simulink library "sm_excv_scene_lib"  (R2023a)
settings: Solver=VariableStepAuto  StartTime=0.0  StopTime=10.0  RelTol=1e-3
undefined symbols (not defined in the file): B1, B2, B3, B4, B5, B6, B7, B8, Excv, L1, L2, L3, L4, L5, L6, L7, L8, L9, Road, S1, S2, Scene, Scene_Data, SceneData, X, Y, Z
libraries: sm_lib x65, sm_tracked_vehicle_lib x47, $bdroot x45, nesl_utility x10
(part 3 of 3)

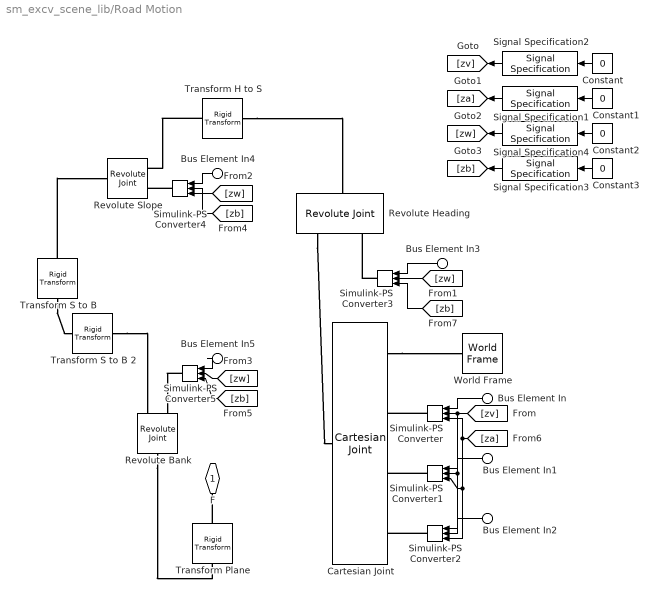
== system sm_excv_scene_lib/Road Motion ==
  Bus Element In : Inport  PortName=Road  Element=px
  Bus Element In1 : Inport  PortName=Road  Element=py
  Bus Element In2 : Inport  PortName=Road  Element=pz
  Bus Element In3 : Inport  PortName=Road  Element=qz
  Bus Element In4 : Inport  PortName=Road  Element=qy
  Bus Element In5 : Inport  PortName=Road  Element=qx
  Cartesian Joint : sm_lib/Joints/Cartesian Joint  JointMode=Normal  SenseConstraintForce=off  SenseConstraintForceX=off  SenseConstraintForceY=off  SenseConstraintForceZ=off  SenseConstraintTorque=off  SenseConstraintTorqueX=off  SenseConstraintTorqueY=off  SenseConstraintTorqueZ=off  SenseTotalForce=off  SenseTotalForceX=off  SenseTotalForceY=off  SenseTotalForceZ=off  SenseTotalTorque=off  SenseTotalTorqueX=off  SenseTotalTorqueY=off  SenseTotalTorqueZ=off  CompositeWrenchDir=FollowerOnBase  CompositeWrenchFrame=BaseFrame  PxEquilibriumPosition=0  PxEquilibriumPositionUnits=m  PxSpringStiffness=0  PxSpringStiffnessUnits=N/m  PxDampingCoefficient=0  PxDampingCoefficientUnits=N/(m/s)  PxTorqueActuationMode=ComputedTorque  PxMotionActuationMode=InputMotion  PxSensePosition=off  PxSenseVelocity=off  PxSenseAcceleration=off  PxSenseTorqueForce=off  PxSenseLowerLimitTorqueForce=off  PxSenseUpperLimitTorqueForce=off  PxLowerLimitSpecify=off  PxLowerLimitBound=-1  PxLowerLimitBoundUnits=m  PxLowerLimitStiffness=1e6  PxLowerLimitStiffnessUnits=N/m  PxLowerLimitDamping=1e3  PxLowerLimitDampingUnits=N/(m/s)  PxLowerLimitTransitionRegionWidth=1e-4  PxLowerLimitTransitionRegionWidthUnits=m  PxUpperLimitSpecify=off  PxUpperLimitBound=1  PxUpperLimitBoundUnits=m  PxUpperLimitStiffness=1e6  PxUpperLimitStiffnessUnits=N/m  PxUpperLimitDamping=1e3  PxUpperLimitDampingUnits=N/(m/s)  PxUpperLimitTransitionRegionWidth=1e-4  PxUpperLimitTransitionRegionWidthUnits=m  PxPositionTargetSpecify=off  PxPositionTargetPriority=High  PxPositionTargetValue=0  PxPositionTargetValueUnits=m  PxVelocityTargetSpecify=off  PxVelocityTargetPriority=High  PxVelocityTargetValue=0  PxVelocityTargetValueUnits=m/s  PyEquilibriumPosition=0  PyEquilibriumPositionUnits=m  PySpringStiffness=0  PySpringStiffnessUnits=N/m  PyDampingCoefficient=0  PyDampingCoefficientUnits=N/(m/s)  PyTorqueActuationMode=ComputedTorque  PyMotionActuationMode=InputMotion  PySensePosition=off  PySenseVelocity=off  PySenseAcceleration=off  PySenseTorqueForce=off  PySenseLowerLimitTorqueForce=off  PySenseUpperLimitTorqueForce=off  PyLowerLimitSpecify=off  PyLowerLimitBound=-1  PyLowerLimitBoundUnits=m  PyLowerLimitStiffness=1e6  PyLowerLimitStiffnessUnits=N/m  PyLowerLimitDamping=1e3  PyLowerLimitDampingUnits=N/(m/s)  PyLowerLimitTransitionRegionWidth=1e-4  PyLowerLimitTransitionRegionWidthUnits=m  PyUpperLimitSpecify=off  PyUpperLimitBound=1  PyUpperLimitBoundUnits=m  PyUpperLimitStiffness=1e6  PyUpperLimitStiffnessUnits=N/m  PyUpperLimitDamping=1e3  PyUpperLimitDampingUnits=N/(m/s)  PyUpperLimitTransitionRegionWidth=1e-4  PyUpperLimitTransitionRegionWidthUnits=m  PyPositionTargetSpecify=off  PyPositionTargetPriority=High  PyPositionTargetValue=0  PyPositionTargetValueUnits=m  PyVelocityTargetSpecify=off  PyVelocityTargetPriority=High  PyVelocityTargetValue=0  PyVelocityTargetValueUnits=m/s  PzEquilibriumPosition=0  PzEquilibriumPositionUnits=m  PzSpringStiffness=0  PzSpringStiffnessUnits=N/m  PzDampingCoefficient=0  PzDampingCoefficientUnits=N/(m/s)  PzTorqueActuationMode=ComputedTorque  PzMotionActuationMode=InputMotion  PzSensePosition=off  PzSenseVelocity=off  PzSenseAcceleration=off  PzSenseTorqueForce=off  PzSenseLowerLimitTorqueForce=off  PzSenseUpperLimitTorqueForce=off  PzLowerLimitSpecify=off  PzLowerLimitBound=-1  PzLowerLimitBoundUnits=m  PzLowerLimitStiffness=1e6  PzLowerLimitStiffnessUnits=N/m  PzLowerLimitDamping=1e3  PzLowerLimitDampingUnits=N/(m/s)  PzLowerLimitTransitionRegionWidth=1e-4  PzLowerLimitTransitionRegionWidthUnits=m  PzUpperLimitSpecify=off  PzUpperLimitBound=1  PzUpperLimitBoundUnits=m  PzUpperLimitStiffness=1e6  PzUpperLimitStiffnessUnits=N/m  PzUpperLimitDamping=1e3  PzUpperLimitDampingUnits=N/(m/s)  PzUpperLimitTransitionRegionWidth=1e-4  PzUpperLimitTransitionRegionWidthUnits=m  PzPositionTargetSpecify=off  PzPositionTargetPriority=High  PzPositionTargetValue=0  PzPositionTargetValueUnits=m  PzVelocityTargetSpecify=off  PzVelocityTargetPriority=High  PzVelocityTargetValue=0  PzVelocityTargetValueUnits=m/s
  Constant{,1..3} (4 alike) : Constant  Value=0
  Revolute Heading : sm_lib/Joints/Revolute Joint  JointMode=Normal  SenseConstraintForce=off  SenseConstraintForceX=off  SenseConstraintForceY=off  SenseConstraintForceZ=off  SenseConstraintTorque=off  SenseConstraintTorqueX=off  SenseConstraintTorqueY=off  SenseConstraintTorqueZ=off  SenseTotalForce=off  SenseTotalForceX=off  SenseTotalForceY=off  SenseTotalForceZ=off  SenseTotalTorque=off  SenseTotalTorqueX=off  SenseTotalTorqueY=off  SenseTotalTorqueZ=off  CompositeWrenchDir=FollowerOnBase  CompositeWrenchFrame=BaseFrame  EquilibriumPosition=0  EquilibriumPositionUnits=deg  SpringStiffness=0  SpringStiffnessUnits=N*m/deg  DampingCoefficient=0  DampingCoefficientUnits=N*m/(deg/s)  TorqueActuationMode=ComputedTorque  MotionActuationMode=InputMotion  SensePosition=off  SenseVelocity=off  SenseAcceleration=off  SenseTorqueForce=off  SenseLowerLimitTorqueForce=off  SenseUpperLimitTorqueForce=off  LowerLimitSpecify=off  LowerLimitBound=-90  LowerLimitBoundUnits=deg  LowerLimitStiffness=1e4  LowerLimitStiffnessUnits=N*m/deg  LowerLimitDamping=10  LowerLimitDampingUnits=N*m/(deg/s)  LowerLimitTransitionRegionWidth=0.1  LowerLimitTransitionRegionWidthUnits=deg  UpperLimitSpecify=off  UpperLimitBound=90  UpperLimitBoundUnits=deg  UpperLimitStiffness=1e4  UpperLimitStiffnessUnits=N*m/deg  UpperLimitDamping=10  UpperLimitDampingUnits=N*m/(deg/s)  UpperLimitTransitionRegionWidth=0.1  UpperLimitTransitionRegionWidthUnits=deg  PositionTargetSpecify=off  PositionTargetPriority=High  PositionTargetValue=0  PositionTargetValueUnits=deg  VelocityTargetSpecify=off  VelocityTargetPriority=High  VelocityTargetValue=0  VelocityTargetValueUnits=deg/s
  Revolute Slope : sm_lib/Joints/Revolute Joint  JointMode=Normal  SenseConstraintForce=off  SenseConstraintForceX=off  SenseConstraintForceY=off  SenseConstraintForceZ=off  SenseConstraintTorque=off  SenseConstraintTorqueX=off  SenseConstraintTorqueY=off  SenseConstraintTorqueZ=off  SenseTotalForce=off  SenseTotalForceX=off  SenseTotalForceY=off  SenseTotalForceZ=off  SenseTotalTorque=off  SenseTotalTorqueX=off  SenseTotalTorqueY=off  SenseTotalTorqueZ=off  CompositeWrenchDir=FollowerOnBase  CompositeWrenchFrame=BaseFrame  EquilibriumPosition=0  EquilibriumPositionUnits=deg  SpringStiffness=0  SpringStiffnessUnits=N*m/deg  DampingCoefficient=0  DampingCoefficientUnits=N*m/(deg/s)  TorqueActuationMode=ComputedTorque  MotionActuationMode=InputMotion  SensePosition=off  SenseVelocity=off  SenseAcceleration=off  SenseTorqueForce=off  SenseLowerLimitTorqueForce=off  SenseUpperLimitTorqueForce=off  LowerLimitSpecify=off  LowerLimitBound=-90  LowerLimitBoundUnits=deg  LowerLimitStiffness=1e4  LowerLimitStiffnessUnits=N*m/deg  LowerLimitDamping=10  LowerLimitDampingUnits=N*m/(deg/s)  LowerLimitTransitionRegionWidth=0.1  LowerLimitTransitionRegionWidthUnits=deg  UpperLimitSpecify=off  UpperLimitBound=90  UpperLimitBoundUnits=deg  UpperLimitStiffness=1e4  UpperLimitStiffnessUnits=N*m/deg  UpperLimitDamping=10  UpperLimitDampingUnits=N*m/(deg/s)  UpperLimitTransitionRegionWidth=0.1  UpperLimitTransitionRegionWidthUnits=deg  PositionTargetSpecify=off  PositionTargetPriority=High  PositionTargetValue=0  PositionTargetValueUnits=deg  VelocityTargetSpecify=off  VelocityTargetPriority=High  VelocityTargetValue=0  VelocityTargetValueUnits=deg/s
  Revolute Bank : sm_lib/Joints/Revolute Joint  JointMode=Normal  SenseConstraintForce=off  SenseConstraintForceX=off  SenseConstraintForceY=off  SenseConstraintForceZ=off  SenseConstraintTorque=off  SenseConstraintTorqueX=off  SenseConstraintTorqueY=off  SenseConstraintTorqueZ=off  SenseTotalForce=off  SenseTotalForceX=off  SenseTotalForceY=off  SenseTotalForceZ=off  SenseTotalTorque=off  SenseTotalTorqueX=off  SenseTotalTorqueY=off  SenseTotalTorqueZ=off  CompositeWrenchDir=FollowerOnBase  CompositeWrenchFrame=BaseFrame  EquilibriumPosition=0  EquilibriumPositionUnits=deg  SpringStiffness=0  SpringStiffnessUnits=N*m/deg  DampingCoefficient=0  DampingCoefficientUnits=N*m/(deg/s)  TorqueActuationMode=ComputedTorque  MotionActuationMode=InputMotion  SensePosition=off  SenseVelocity=off  SenseAcceleration=off  SenseTorqueForce=off  SenseLowerLimitTorqueForce=off  SenseUpperLimitTorqueForce=off  LowerLimitSpecify=off  LowerLimitBound=-90  LowerLimitBoundUnits=deg  LowerLimitStiffness=1e4  LowerLimitStiffnessUnits=N*m/deg  LowerLimitDamping=10  LowerLimitDampingUnits=N*m/(deg/s)  LowerLimitTransitionRegionWidth=0.1  LowerLimitTransitionRegionWidthUnits=deg  UpperLimitSpecify=off  UpperLimitBound=90  UpperLimitBoundUnits=deg  UpperLimitStiffness=1e4  UpperLimitStiffnessUnits=N*m/deg  UpperLimitDamping=10  UpperLimitDampingUnits=N*m/(deg/s)  UpperLimitTransitionRegionWidth=0.1  UpperLimitTransitionRegionWidthUnits=deg  PositionTargetSpecify=off  PositionTargetPriority=High  PositionTargetValue=0  PositionTargetValueUnits=deg  VelocityTargetSpecify=off  VelocityTargetPriority=High  VelocityTargetValue=0  VelocityTargetValueUnits=deg/s
  Signal Specification1 : SignalSpecification  Unit=m/s^2
  Signal Specification2 : SignalSpecification  Unit=m/s
  Signal Specification3 : SignalSpecification  Unit=rad/s^2
  Signal Specification4 : SignalSpecification  Unit=rad/s
  Simulink-PS Converter : nesl_utility/Simulink-PS Converter  PhysicalDomain=network_engine_domain  SubClassName=ps_input  LeftPortType=input  RightPortType=output  PseudoPeriodic=off  Frequencies=[]  NoiseDistribution=none  NoiseParameters=[]  Unit=m  AffineConversion=off  FilteringAndDerivatives=provide  SimscapeFilterOrder=1  InputFilterTimeConstant=0.001  UdotUserProvided=2
  Simulink-PS Converter1 : nesl_utility/Simulink-PS Converter  PhysicalDomain=network_engine_domain  SubClassName=ps_input  LeftPortType=input  RightPortType=output  PseudoPeriodic=off  Frequencies=[]  NoiseDistribution=none  NoiseParameters=[]  Unit=m  AffineConversion=off  FilteringAndDerivatives=provide  SimscapeFilterOrder=1  InputFilterTimeConstant=0.001  UdotUserProvided=2
  Simulink-PS Converter2 : nesl_utility/Simulink-PS Converter  PhysicalDomain=network_engine_domain  SubClassName=ps_input  LeftPortType=input  RightPortType=output  PseudoPeriodic=off  Frequencies=[]  NoiseDistribution=none  NoiseParameters=[]  Unit=m  AffineConversion=off  FilteringAndDerivatives=provide  SimscapeFilterOrder=1  InputFilterTimeConstant=0.001  UdotUserProvided=2
  Simulink-PS Converter3 : nesl_utility/Simulink-PS Converter  PhysicalDomain=network_engine_domain  SubClassName=ps_input  LeftPortType=input  RightPortType=output  PseudoPeriodic=off  Frequencies=[]  NoiseDistribution=none  NoiseParameters=[]  Unit=rad  AffineConversion=off  FilteringAndDerivatives=provide  SimscapeFilterOrder=1  InputFilterTimeConstant=0.001  UdotUserProvided=2
  Simulink-PS Converter4 : nesl_utility/Simulink-PS Converter  PhysicalDomain=network_engine_domain  SubClassName=ps_input  LeftPortType=input  RightPortType=output  PseudoPeriodic=off  Frequencies=[]  NoiseDistribution=none  NoiseParameters=[]  Unit=rad  AffineConversion=off  FilteringAndDerivatives=provide  SimscapeFilterOrder=1  InputFilterTimeConstant=0.001  UdotUserProvided=2
  Simulink-PS Converter5 : nesl_utility/Simulink-PS Converter  PhysicalDomain=network_engine_domain  SubClassName=ps_input  LeftPortType=input  RightPortType=output  PseudoPeriodic=off  Frequencies=[]  NoiseDistribution=none  NoiseParameters=[]  Unit=rad  AffineConversion=off  FilteringAndDerivatives=provide  SimscapeFilterOrder=1  InputFilterTimeConstant=0.001  UdotUserProvided=2
  Transform H to S : sm_lib/Frames and Transforms/Rigid Transform  TranslationMethod=None  TranslationStandardOffset=0  TranslationStandardOffsetUnits=m  TranslationStandardAxis=+Z  TranslationCartesianOffset=[0 0 0]  TranslationCartesianOffsetUnits=m  TranslationROffset=0  TranslationROffsetUnits=m  TranslationZOffset=0  TranslationZOffsetUnits=m  TranslationThetaOffset=0  TranslationThetaOffsetUnits=deg  RotationMethod=AlignedAxes  RotationAngleUnits=deg  RotationStandardAxis=+Z  RotationAngle=0.0  RotationArbitraryAxis=[0 0 1]  FollAlignAxisA=+Z  BaseAlignAxisA=+Y  FollAlignAxisB=+X  BaseAlignAxisB=+X  RotationSequenceAxes=FollowerAxes  RotationSequence=XYX  RotationSequenceAngles=[0 0 0]  RotationSequenceAnglesUnits=deg  RotationMatrix=[1 0 0; 0 1 0; 0 0 1]  Quaternion=[1 0 0 0]
  Transform Plane : sm_lib/Frames and Transforms/Rigid Transform  TranslationMethod=None  TranslationStandardOffset=0  TranslationStandardOffsetUnits=m  TranslationStandardAxis=+Z  TranslationCartesianOffset=[0 0 0]  TranslationCartesianOffsetUnits=m  TranslationROffset=0  TranslationROffsetUnits=m  TranslationZOffset=0  TranslationZOffsetUnits=m  TranslationThetaOffset=0  TranslationThetaOffsetUnits=deg  RotationMethod=AlignedAxes  RotationAngleUnits=deg  RotationStandardAxis=+Z  RotationAngle=0.0  RotationArbitraryAxis=[0 0 1]  FollAlignAxisA=+Z  BaseAlignAxisA=-X  FollAlignAxisB=+Y  BaseAlignAxisB=+Y  RotationSequenceAxes=FollowerAxes  RotationSequence=XYX  RotationSequenceAngles=[0 0 0]  RotationSequenceAnglesUnits=deg  RotationMatrix=[1 0 0; 0 1 0; 0 0 1]  Quaternion=[1 0 0 0]
  Transform S to B : sm_lib/Frames and Transforms/Rigid Transform  TranslationMethod=None  TranslationStandardOffset=0  TranslationStandardOffsetUnits=m  TranslationStandardAxis=+Z  TranslationCartesianOffset=[0 0 0]  TranslationCartesianOffsetUnits=m  TranslationROffset=0  TranslationROffsetUnits=m  TranslationZOffset=0  TranslationZOffsetUnits=m  TranslationThetaOffset=0  TranslationThetaOffsetUnits=deg  RotationMethod=AlignedAxes  RotationAngleUnits=deg  RotationStandardAxis=+Z  RotationAngle=0.0  RotationArbitraryAxis=[0 0 1]  FollAlignAxisA=+Z  BaseAlignAxisA=-Y  FollAlignAxisB=+X  BaseAlignAxisB=+X  RotationSequenceAxes=FollowerAxes  RotationSequence=XYX  RotationSequenceAngles=[0 0 0]  RotationSequenceAnglesUnits=deg  RotationMatrix=[1 0 0; 0 1 0; 0 0 1]  Quaternion=[1 0 0 0]
  Transform S to B 2 : sm_lib/Frames and Transforms/Rigid Transform  TranslationMethod=None  TranslationStandardOffset=0  TranslationStandardOffsetUnits=m  TranslationStandardAxis=+Z  TranslationCartesianOffset=[0 0 0]  TranslationCartesianOffsetUnits=m  TranslationROffset=0  TranslationROffsetUnits=m  TranslationZOffset=0  TranslationZOffsetUnits=m  TranslationThetaOffset=0  TranslationThetaOffsetUnits=deg  RotationMethod=AlignedAxes  RotationAngleUnits=deg  RotationStandardAxis=+Z  RotationAngle=0.0  RotationArbitraryAxis=[0 0 1]  FollAlignAxisA=+Z  BaseAlignAxisA=+X  FollAlignAxisB=+Y  BaseAlignAxisB=+Y  RotationSequenceAxes=FollowerAxes  RotationSequence=XYX  RotationSequenceAngles=[0 0 0]  RotationSequenceAnglesUnits=deg  RotationMatrix=[1 0 0; 0 1 0; 0 0 1]  Quaternion=[1 0 0 0]
  World Frame : sm_lib/Frames and Transforms/World Frame
  F : PMIOPort  Side=Right
  wires:
  Constant2/1 -> Signal Specification4/1
  Constant3/1 -> Signal Specification3/1
  Signal Specification4/1 -> [zw]
  Signal Specification3/1 -> [zb]
  Signal Specification1/1 -> [za]
  Signal Specification2/1 -> [zv]
  [zb] -> Simulink-PS Converter3/3
  [za] -> Simulink-PS Converter1/3, Simulink-PS Converter2/3, Simulink-PS Converter/3
  [zb] -> Simulink-PS Converter5/3
  [zb] -> Simulink-PS Converter4/3
  Constant1/1 -> Signal Specification1/1
  [zw] -> Simulink-PS Converter3/2
  [zw] -> Simulink-PS Converter5/2
  [zv] -> Simulink-PS Converter/2, Simulink-PS Converter1/2, Simulink-PS Converter2/2
  [zw] -> Simulink-PS Converter4/2
  Constant/1 -> Signal Specification2/1
  Bus Element In5/1 -> Simulink-PS Converter5/1
  Bus Element In4/1 -> Simulink-PS Converter4/1
  Bus Element In3/1 -> Simulink-PS Converter3/1
  Bus Element In2/1 -> Simulink-PS Converter2/1
  Bus Element In1/1 -> Simulink-PS Converter1/1
  Bus Element In/1 -> Simulink-PS Converter/1
  connections:
  Simulink-PS Converter2/RConn1 -- Cartesian Joint/LConn4
  Simulink-PS Converter5/RConn1 -- Revolute Bank/LConn2
  Simulink-PS Converter3/RConn1 -- Revolute Heading/LConn2
  Cartesian Joint/LConn1 -- World Frame/RConn1
  Simulink-PS Converter4/RConn1 -- Revolute Slope/LConn2
  Simulink-PS Converter/RConn1 -- Cartesian Joint/LConn2
  Transform S to B/RConn1 -- Transform S to B 2/LConn1
  Transform S to B 2/RConn1 -- Revolute Bank/LConn1
  Transform S to B/LConn1 -- Revolute Slope/RConn1
  Revolute Heading/LConn1 -- Cartesian Joint/RConn1
  Simulink-PS Converter1/RConn1 -- Cartesian Joint/LConn3
  Transform Plane/RConn1 -- F/RConn1
  Revolute Bank/RConn1 -- Transform Plane/LConn1
  Transform H to S/LConn1 -- Revolute Heading/RConn1
  Transform H to S/RConn1 -- Revolute Slope/LConn1

== system sm_excv_scene_lib/Road Profile Left Right ==
  RDF Polyline : Subsystem  mask(Left and Right Paths){road_extr_data_L=RDF_Polyline.Road.extr_data_L, road_extr_data_R=RDF_Polyline.Road.extr_data_R, road_profile_sep=RDF_Polyline.Road.profile_separation, road_w=RDF_Polyline.Road.w, road_x=RDF_Polyline.Road.x, road_z=RDF_Polyline.Road.z, road_yaw=RDF_Polyline.Road.yaw, road_clr=RDF_Polyline.Road.clr, road_opc=RDF_Polyline.Road.opc}
      mask prompts: road_extr_data_L "Road Profile Left [x y] (m)"; road_extr_data_R "Road Profile Right [x y] (m)"; road_profile_sep "Profile Separation (m)"; road_w "Width (m)"; road_x "Offset x (m)"; road_z "Offset z (m)"; road_yaw "Offset yaw (rad)"; road_clr "Color [R G B]"; road_opc "Opacity (0-1)"
      mask help: Creates left and right straightline paths for wheels as an extrusion.
  W : PMIOPort  Side=Left
  connections:
  W/RConn1 -- RDF Polyline/RConn1

== system sm_excv_scene_lib/Road Profile and Grid ==
  Grid : $bdroot/Grid  VariantControl=Grid  grid_x=grid_x  grid_y=grid_y  grid_z=grid_z  grid_line_width=grid_line_width  grid_num_sq_x=grid_num_sq_x  grid_num_sq_y=grid_num_sq_y  grid_clr=grid_clr  plane_clr=plane_clr  grid_opc=grid_opc
  Plateau : $bdroot/Road Profile Left Right  RDF_Polyline=RDF_Polyline
      settings: LibrarySourceBlock=sm_excv_uneven_road_lib/Scene Plateau
  Transform Grid Offset : sm_lib/Frames and Transforms/Rigid Transform  TranslationMethod=Cartesian  TranslationStandardOffset=0  TranslationStandardOffsetUnits=m  TranslationStandardAxis=+X  TranslationCartesianOffset=[grid_x*0.45 0 grid_z_offset]  TranslationCartesianOffsetUnits=m  TranslationROffset=0  TranslationROffsetUnits=m  TranslationZOffset=0  TranslationZOffsetUnits=m  TranslationThetaOffset=0  TranslationThetaOffsetUnits=deg  RotationMethod=None  RotationAngleUnits=deg  RotationStandardAxis=+Z  RotationAngle=0.0  RotationArbitraryAxis=[0 0 1]  FollAlignAxisA=+X  BaseAlignAxisA=+Y  FollAlignAxisB=+Y  BaseAlignAxisB=+Z  RotationSequenceAxes=FollowerAxes  RotationSequence=XYX  RotationSequenceAngles=[0 0 0]  RotationSequenceAnglesUnits=deg  RotationMatrix=[1 0 0; 0 1 0; 0 0 1]  Quaternion=[1 0 0 0]
  B : PMIOPort  Side=Right
  connections:
  B/RConn1 -- Transform Grid Offset/LConn1 -- Plateau/LConn1
  Grid/RConn1 -- Transform Grid Offset/RConn1

== system sm_excv_scene_lib/Rough Road 1 Roller Spheres ==
  mL : Inport
  Rough Road : $bdroot/Road Profile and Grid  VariantControl=Plateau  RDF_Polyline=Scene.Rough_Road  grid_z_offset=-0.2  grid_x=Scene.Grid.length*0.5  grid_y=Scene.Grid.width*0.01  grid_z=Scene.Grid.depth  grid_line_width=Scene.Grid.linewidth  grid_num_sq_x=Scene.Grid.numsquaresx*0.5  grid_num_sq_y=Scene.Grid.numsquaresy*0.01  plane_clr=Scene.Grid.linecolor  grid_clr=Scene.Grid.planecolor  grid_opc=1
  Rough Road L : $bdroot/Wheel Center to Patch 2x Roller Set  road_pz_x=Scene.Rough_Road.Road.pzLUT.px  road_pz_z=Scene.Rough_Road.Road.pzLUT.pz(:,1)  road_qy_x=Scene.Rough_Road.Road.qyLUT.px  road_qy_qy=Scene.Rough_Road.Road.qyLUT.qy(:,1)  tfilter=0.01  NormalStiffness=Scene.Contact.Terrain.K  NormalDamping=Scene.Contact.Terrain.B  NormalTransitionRegionWidth=Scene.Contact.Terrain.TW  CoefficientOfDynamicFriction=Scene.Contact.Terrain.mud  CoefficientOfStaticFriction=Scene.Contact.Terrain.mus  FrictionalCriticalVelocity=Scene.Contact.Terrain.CV  patch_x=Scene.Patch.w  patch_y=Scene.Patch.l  patch_clr=Scene.Patch.clr  patch_opc=Scene.Patch.opc
      settings: LibrarySourceBlock=sm_excv_uneven_road_lib/Rollers Rough Road1
  L : PMIOPort  Side=Right
  W : PMIOPort  Port=2  Side=Right
  wires:
  mL/1 -> Rough Road L/1
  connections:
  Rough Road/RConn1 -- W/RConn1
  Rough Road L/RConn1 -- L/RConn1

== system sm_excv_scene_lib/Rough Road 2 Rollers Spheres ==
  mL : Inport
  mR : Inport  Port=2
  Rough Road : $bdroot/Road Profile and Grid  VariantControl=Plateau  RDF_Polyline=Scene.Rough_Road  grid_z_offset=-0.2  grid_x=Scene.Grid.length*0.5  grid_y=Scene.Grid.width*0.01  grid_z=Scene.Grid.depth  grid_line_width=Scene.Grid.linewidth  grid_num_sq_x=Scene.Grid.numsquaresx*0.5  grid_num_sq_y=Scene.Grid.numsquaresy*0.01  plane_clr=Scene.Grid.linecolor  grid_clr=Scene.Grid.planecolor  grid_opc=1
  Rough Road L : $bdroot/Wheel Center to Patch 2x Roller Set  road_pz_x=Scene.Rough_Road.Road.pzLUT.px  road_pz_z=Scene.Rough_Road.Road.pzLUT.pz(:,1)  road_qy_x=Scene.Rough_Road.Road.qyLUT.px  road_qy_qy=Scene.Rough_Road.Road.qyLUT.qy(:,1)  tfilter=0.01  NormalStiffness=Scene.Contact.Terrain.K  NormalDamping=Scene.Contact.Terrain.B  NormalTransitionRegionWidth=Scene.Contact.Terrain.TW  CoefficientOfDynamicFriction=Scene.Contact.Terrain.mud  CoefficientOfStaticFriction=Scene.Contact.Terrain.mus  FrictionalCriticalVelocity=Scene.Contact.Terrain.CV  patch_x=Scene.Patch.w  patch_y=Scene.Patch.l  patch_clr=Scene.Patch.clr  patch_opc=Scene.Patch.opc
      settings: LibrarySourceBlock=sm_excv_uneven_road_lib/Rollers Rough Road1
  Rough Road R : $bdroot/Wheel Center to Patch 2x Roller Set  road_pz_x=Scene.Rough_Road.Road.pzLUT.px  road_pz_z=Scene.Rough_Road.Road.pzLUT.pz(:,2)  road_qy_x=Scene.Rough_Road.Road.qyLUT.px  road_qy_qy=Scene.Rough_Road.Road.qyLUT.qy(:,2)  tfilter=0.01  NormalStiffness=Scene.Contact.Terrain.K  NormalDamping=Scene.Contact.Terrain.B  NormalTransitionRegionWidth=Scene.Contact.Terrain.TW  CoefficientOfDynamicFriction=Scene.Contact.Terrain.mud  CoefficientOfStaticFriction=Scene.Contact.Terrain.mus  FrictionalCriticalVelocity=Scene.Contact.Terrain.CV  patch_x=Scene.Patch.w  patch_y=Scene.Patch.l  patch_clr=Scene.Patch.clr  patch_opc=Scene.Patch.opc
      settings: LibrarySourceBlock=sm_excv_uneven_road_lib/Rollers Rough Road1
  L : PMIOPort  Side=Right
  W : PMIOPort  Port=2  Side=Right
  R : PMIOPort  Port=3  Side=Right
  wires:
  mR/1 -> Rough Road R/1
  mL/1 -> Rough Road L/1
  connections:
  Rough Road L/RConn1 -- L/RConn1
  Rough Road/RConn1 -- W/RConn1
  Rough Road R/RConn1 -- R/RConn1

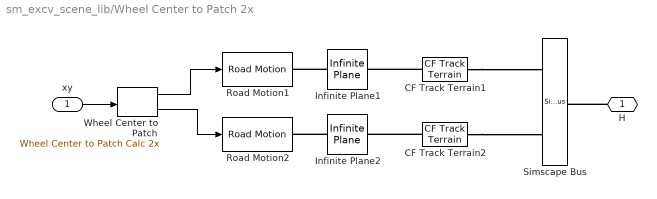
== system sm_excv_scene_lib/Wheel Center to Patch 2x ==
  xy : Inport
  CF Track Terrain1 : sm_tracked_vehicle_lib/CF Track Terrain  NormalStiffness=NormalStiffness  NormalDamping=NormalDamping  NormalTransitionRegionWidth=NormalTransitionRegionWidth  CoefficientOfDynamicFriction=CoefficientOfDynamicFriction  CoefficientOfStaticFriction=CoefficientOfStaticFriction  FrictionalCriticalVelocity=FrictionalCriticalVelocity
  CF Track Terrain2 : sm_tracked_vehicle_lib/CF Track Terrain  NormalStiffness=NormalStiffness  NormalDamping=NormalDamping  NormalTransitionRegionWidth=NormalTransitionRegionWidth  CoefficientOfDynamicFriction=CoefficientOfDynamicFriction  CoefficientOfStaticFriction=CoefficientOfStaticFriction  FrictionalCriticalVelocity=FrictionalCriticalVelocity
  Infinite Plane1 : sm_lib/Curves and Surfaces/Infinite Plane  GraphicType=Rectangle  GraphicPlaneWidth=patch_x  GraphicPlaneWidthUnits=m  GraphicPlaneHeight=patch_y  GraphicPlaneHeightUnits=m  GraphicVisPropType=SimpleVisualProperties  GraphicDiffuseColor=patch_clr  GraphicOpacity=patch_opc  GraphicSpecularColor=[0.5 0.5 0.5 1.0]  GraphicAmbientColor=[0.15 0.15 0.15 1.0]  GraphicEmissiveColor=[0.0 0.0 0.0 1.0]  GraphicShininess=75
  Infinite Plane2 : sm_lib/Curves and Surfaces/Infinite Plane  GraphicType=Rectangle  GraphicPlaneWidth=patch_x  GraphicPlaneWidthUnits=m  GraphicPlaneHeight=patch_y  GraphicPlaneHeightUnits=m  GraphicVisPropType=SimpleVisualProperties  GraphicDiffuseColor=patch_clr  GraphicOpacity=patch_opc  GraphicSpecularColor=[0.5 0.5 0.5 1.0]  GraphicAmbientColor=[0.15 0.15 0.15 1.0]  GraphicEmissiveColor=[0.0 0.0 0.0 1.0]  GraphicShininess=75
  Road Motion1 : $bdroot/Road Motion  SystemSampleTime=-1  VariantActivationTime=update diagram  Latency=0  AutoFrameSizeCalculation=off
  Road Motion2 : $bdroot/Road Motion  SystemSampleTime=-1  VariantActivationTime=update diagram  Latency=0  AutoFrameSizeCalculation=off
  Simscape Bus : SimscapeBus  HierarchyStrings=S1;S2
  Wheel Center to Patch : $bdroot/Wheel Center to Patch Calc 2x  road_pz_x=road_pz_x  road_pz_z=road_pz_z  road_qy_x=road_qy_x  road_qy_qy=road_qy_qy  tfilter=tfilter
      settings: LibrarySourceBlock=|
      | sm_excv_uneven_road_lib/Patch Position
      | Rough Road1
  H : PMIOPort  Side=Right
  wires:
  Wheel Center to Patch/1 -> Road Motion1/1
  Wheel Center to Patch/2 -> Road Motion2/1
  xy/1 -> Wheel Center to Patch/1
  connections:
  CF Track Terrain2/RConn1 -- Simscape Bus/LConn2
  CF Track Terrain1/RConn1 -- Simscape Bus/LConn1
  H/RConn1 -- Simscape Bus/RConn1
  CF Track Terrain2/LConn1 -- Infinite Plane2/RConn1
  Infinite Plane2/LConn1 -- Road Motion2/RConn1
  CF Track Terrain1/LConn1 -- Infinite Plane1/RConn1
  Infinite Plane1/LConn1 -- Road Motion1/RConn1

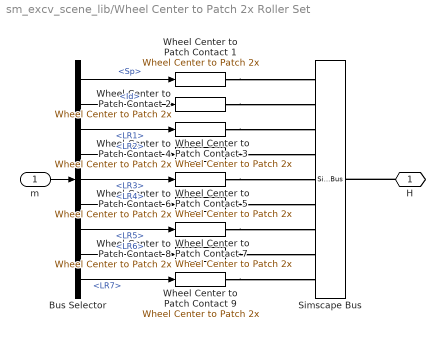
== system sm_excv_scene_lib/Wheel Center to Patch 2x Roller Set ==
  m : Inport
  Bus Selector : BusSelector  OutputSignals=Underc.Sp,Underc.Id,Underc.LR1,Underc.LR2,Underc.LR3,Underc.LR4,Underc.LR5,Underc.LR6,Underc.LR7
  Simscape Bus : SimscapeBus  HierarchyStrings=L1;L2;L3;L4;L5;L6;L7;L8;L9
  Wheel Center to Patch Contact {1..9} (9 alike) : $bdroot/Wheel Center to Patch 2x  road_pz_x=road_pz_x  road_pz_z=road_pz_z  road_qy_x=road_qy_x  road_qy_qy=road_qy_qy  tfilter=tfilter  patch_clr=patch_clr  patch_opc=patch_opc  patch_x=patch_x  patch_y=patch_y  NormalStiffness=NormalStiffness  NormalDamping=NormalDamping  NormalTransitionRegionWidth=NormalTransitionRegionWidth  CoefficientOfDynamicFriction=CoefficientOfDynamicFriction  CoefficientOfStaticFriction=CoefficientOfStaticFriction  FrictionalCriticalVelocity=FrictionalCriticalVelocity
      settings: LibrarySourceBlock=sm_excv_uneven_road_lib/Rough Road 1 Roller1
  H : PMIOPort  Side=Right
  wires:
  m/1 -> Bus Selector/1
  Bus Selector/1 -> Wheel Center to Patch Contact 1/1  "<Sp>"
  Bus Selector/6 -> Wheel Center to Patch Contact 6/1  "<LR4>"
  Bus Selector/7 -> Wheel Center to Patch Contact 7/1  "<LR5>"
  Bus Selector/2 -> Wheel Center to Patch Contact 2/1  "<Id>"
  Bus Selector/5 -> Wheel Center to Patch Contact 5/1  "<LR3>"
  Bus Selector/4 -> Wheel Center to Patch Contact 4/1  "<LR2>"
  Bus Selector/8 -> Wheel Center to Patch Contact 8/1  "<LR6>"
  Bus Selector/9 -> Wheel Center to Patch Contact 9/1  "<LR7>"
  Bus Selector/3 -> Wheel Center to Patch Contact 3/1  "<LR1>"
  connections:
  H/RConn1 -- Simscape Bus/RConn1
  Wheel Center to Patch Contact 4/RConn1 -- Simscape Bus/LConn4
  Wheel Center to Patch Contact 5/RConn1 -- Simscape Bus/LConn5
  Wheel Center to Patch Contact 2/RConn1 -- Simscape Bus/LConn2
  Wheel Center to Patch Contact 9/RConn1 -- Simscape Bus/LConn9
  Wheel Center to Patch Contact 6/RConn1 -- Simscape Bus/LConn6
  Wheel Center to Patch Contact 1/RConn1 -- Simscape Bus/LConn1
  Wheel Center to Patch Contact 7/RConn1 -- Simscape Bus/LConn7
  Wheel Center to Patch Contact 3/RConn1 -- Simscape Bus/LConn3
  Wheel Center to Patch Contact 8/RConn1 -- Simscape Bus/LConn8

== system sm_excv_scene_lib/Wheel Center to Patch Calc ==
  note: This implementation only varies road height and pitch along World x-axis.
  x : Inport
  y : Inport  Port=2
  1-D Lookup Table pitch : Lookup_n-D  NumberOfTableDimensions=1  BreakpointsForDimension1=road_qy_x  Table=road_qy_qy  InterpMethod=Akima spline  InternalRulePriority=Speed  RndMeth=Simplest
  1-D Lookup Table pz : Lookup_n-D  NumberOfTableDimensions=1  BreakpointsForDimension1=road_pz_x  Table=road_pz_z  InterpMethod=Akima spline  InternalRulePriority=Speed  RndMeth=Simplest
  Bus Creator1 : BusCreator  Inputs=6
  Constant : Constant  Value=0
  Constant2 : Constant  Value=0
  R : Outport
  wires:
  x/1 -> Bus Creator1/1, 1-D Lookup Table pz/1, 1-D Lookup Table pitch/1  "px"
  y/1 -> Bus Creator1/2  "py"
  Constant/1 -> Bus Creator1/4  "qx"
  Constant2/1 -> Bus Creator1/6  "qz"
  Bus Creator1/1 -> R/1
  1-D Lookup Table pitch/1 -> Bus Creator1/5  "qy"
  1-D Lookup Table pz/1 -> Bus Creator1/3  "pz"

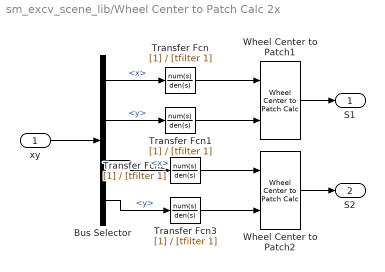
== system sm_excv_scene_lib/Wheel Center to Patch Calc 2x ==
  xy : Inport
  Bus Selector : BusSelector  OutputSignals=S1.x,S1.y,S2.x,S2.y
  Transfer Fcn{,1..3} (4 alike) : TransferFcn  Denominator=[tfilter 1]
  Wheel Center to Patch1 : $bdroot/Wheel Center to Patch Calc  road_pz_x=road_pz_x  road_pz_z=road_pz_z  road_qy_x=road_qy_x  road_qy_qy=road_qy_qy
      settings: LibrarySourceBlock=sm_excv_uneven_road_lib/Rough Road Calc1
  Wheel Center to Patch2 : $bdroot/Wheel Center to Patch Calc  road_pz_x=road_pz_x  road_pz_z=road_pz_z  road_qy_x=road_qy_x  road_qy_qy=road_qy_qy
      settings: LibrarySourceBlock=sm_excv_uneven_road_lib/Rough Road Calc1
  S1 : Outport
  S2 : Outport  Port=2
  wires:
  Transfer Fcn3/1 -> Wheel Center to Patch2/2
  Transfer Fcn2/1 -> Wheel Center to Patch2/1
  Transfer Fcn1/1 -> Wheel Center to Patch1/2
  Transfer Fcn/1 -> Wheel Center to Patch1/1
  Bus Selector/4 -> Transfer Fcn3/1  "<y>"
  Bus Selector/3 -> Transfer Fcn2/1  "<x>"
  Wheel Center to Patch2/1 -> S2/1
  Wheel Center to Patch1/1 -> S1/1
  xy/1 -> Bus Selector/1
  Bus Selector/1 -> Transfer Fcn/1  "<x>"
  Bus Selector/2 -> Transfer Fcn1/1  "<y>"

== system sm_excv_scene_lib/Road Profile Left Right/RDF Polyline ==
  Profile Left : sm_lib/Body Elements/Extruded Solid  GraphicAmbientColor=[0.15 0.15 0.15 1.0]  BasedOnType=Density  CenterOfMass=[0 0 0]  CenterOfMassUnits=m  GraphicDiffuseColor=road_clr  ExportConvexHullGeometry=off  ExtrusionCrossSection=road_extr_data_L  ExtrusionCrossSectionUnits=m  Density=1000  DensityUnits=kg/m^3  DoExposeReferenceFrame=on  GraphicEmissiveColor=[0.0 0.0 0.0 1.0]  ExportEntireGeometry=off  ExtrusionLength=road_w  ExtrusionLengthUnits=m  ExtrusionType=General  SerializedFrames=<Frames/>  MarkerShape=Sphere  MarkerSize=10  GraphicType=FromGeometry  InertiaType=CalculateFromGeometry  Mass=1  MassUnits=kg  MomentsOfInertia=[1 1 1]  MomentsOfInertiaUnits=kg*m^2  PolygonNumSides=3  GraphicOpacity=road_opc  PolygonOuterRadius=1  PolygonOuterRadiusUnits=m  ProductsOfInertia=[0 0 0]  ProductsOfInertiaUnits=kg*m^2  GraphicShininess=75  GraphicSpecularColor=[0.5 0.5 0.5 1.0]  GraphicVisPropType=SimpleVisualProperties
  Profile Right : sm_lib/Body Elements/Extruded Solid  GraphicAmbientColor=[0.15 0.15 0.15 1.0]  BasedOnType=Density  CenterOfMass=[0 0 0]  CenterOfMassUnits=m  GraphicDiffuseColor=road_clr  ExportConvexHullGeometry=off  ExtrusionCrossSection=road_extr_data_R  ExtrusionCrossSectionUnits=m  Density=1000  DensityUnits=kg/m^3  DoExposeReferenceFrame=on  GraphicEmissiveColor=[0.0 0.0 0.0 1.0]  ExportEntireGeometry=off  ExtrusionLength=road_w  ExtrusionLengthUnits=m  ExtrusionType=General  SerializedFrames=<Frames/>  MarkerShape=Sphere  MarkerSize=10  GraphicType=FromGeometry  InertiaType=CalculateFromGeometry  Mass=1  MassUnits=kg  MomentsOfInertia=[1 1 1]  MomentsOfInertiaUnits=kg*m^2  PolygonNumSides=3  GraphicOpacity=road_opc  PolygonOuterRadius=1  PolygonOuterRadiusUnits=m  ProductsOfInertia=[0 0 0]  ProductsOfInertiaUnits=kg*m^2  GraphicShininess=75  GraphicSpecularColor=[0.5 0.5 0.5 1.0]  GraphicVisPropType=SimpleVisualProperties
  Transform Left Profile : sm_lib/Frames and Transforms/Rigid Transform  TranslationMethod=StandardAxis  TranslationStandardOffset=road_profile_sep/2  TranslationStandardOffsetUnits=m  TranslationStandardAxis=+Y  TranslationCartesianOffset=[0 0 0]  TranslationCartesianOffsetUnits=m  TranslationROffset=0  TranslationROffsetUnits=m  TranslationZOffset=0  TranslationZOffsetUnits=m  TranslationThetaOffset=0  TranslationThetaOffsetUnits=deg  RotationMethod=None  RotationAngleUnits=rad  RotationStandardAxis=+Z  RotationAngle=0  RotationArbitraryAxis=[0 0 1]  FollAlignAxisA=+X  BaseAlignAxisA=+Y  FollAlignAxisB=+Y  BaseAlignAxisB=+Z  RotationSequenceAxes=FollowerAxes  RotationSequence=XYX  RotationSequenceAngles=[0 0 0]  RotationSequenceAnglesUnits=deg  RotationMatrix=[1 0 0; 0 1 0; 0 0 1]  Quaternion=[1 0 0 0]
  Transform Right Profile : sm_lib/Frames and Transforms/Rigid Transform  TranslationMethod=StandardAxis  TranslationStandardOffset=road_profile_sep/2  TranslationStandardOffsetUnits=m  TranslationStandardAxis=-Y  TranslationCartesianOffset=[0 0 0]  TranslationCartesianOffsetUnits=m  TranslationROffset=0  TranslationROffsetUnits=m  TranslationZOffset=0  TranslationZOffsetUnits=m  TranslationThetaOffset=0  TranslationThetaOffsetUnits=deg  RotationMethod=None  RotationAngleUnits=rad  RotationStandardAxis=+Z  RotationAngle=0  RotationArbitraryAxis=[0 0 1]  FollAlignAxisA=+X  BaseAlignAxisA=+Y  FollAlignAxisB=+Y  BaseAlignAxisB=+Z  RotationSequenceAxes=FollowerAxes  RotationSequence=XYX  RotationSequenceAngles=[0 0 0]  RotationSequenceAnglesUnits=deg  RotationMatrix=[1 0 0; 0 1 0; 0 0 1]  Quaternion=[1 0 0 0]
  Transform Road : sm_lib/Frames and Transforms/Rigid Transform  TranslationMethod=Cartesian  TranslationStandardOffset=0  TranslationStandardOffsetUnits=m  TranslationStandardAxis=+Z  TranslationCartesianOffset=[road_x 0 road_z]  TranslationCartesianOffsetUnits=m  TranslationROffset=0  TranslationROffsetUnits=m  TranslationZOffset=0  TranslationZOffsetUnits=m  TranslationThetaOffset=0  TranslationThetaOffsetUnits=deg  RotationMethod=StandardAxis  RotationAngleUnits=rad  RotationStandardAxis=+Z  RotationAngle=road_yaw  RotationArbitraryAxis=[0 0 1]  FollAlignAxisA=+X  BaseAlignAxisA=+Y  FollAlignAxisB=+Y  BaseAlignAxisB=+Z  RotationSequenceAxes=FollowerAxes  RotationSequence=XYX  RotationSequenceAngles=[0 0 0]  RotationSequenceAnglesUnits=deg  RotationMatrix=[1 0 0; 0 1 0; 0 0 1]  Quaternion=[1 0 0 0]
  Transform Z to Y Left : sm_lib/Frames and Transforms/Rigid Transform  TranslationMethod=None  TranslationStandardOffset=0  TranslationStandardOffsetUnits=m  TranslationStandardAxis=+Z  TranslationCartesianOffset=[0 0 0]  TranslationCartesianOffsetUnits=m  TranslationROffset=0  TranslationROffsetUnits=m  TranslationZOffset=0  TranslationZOffsetUnits=m  TranslationThetaOffset=0  TranslationThetaOffsetUnits=deg  RotationMethod=StandardAxis  RotationAngleUnits=deg  RotationStandardAxis=+X  RotationAngle=90  RotationArbitraryAxis=[0 0 1]  FollAlignAxisA=+X  BaseAlignAxisA=+Y  FollAlignAxisB=+Y  BaseAlignAxisB=+Z  RotationSequenceAxes=FollowerAxes  RotationSequence=XYX  RotationSequenceAngles=[0 0 0]  RotationSequenceAnglesUnits=deg  RotationMatrix=[1 0 0; 0 1 0; 0 0 1]  Quaternion=[1 0 0 0]
  Transform Z to Y Right : sm_lib/Frames and Transforms/Rigid Transform  TranslationMethod=None  TranslationStandardOffset=0  TranslationStandardOffsetUnits=m  TranslationStandardAxis=+Z  TranslationCartesianOffset=[0 0 0]  TranslationCartesianOffsetUnits=m  TranslationROffset=0  TranslationROffsetUnits=m  TranslationZOffset=0  TranslationZOffsetUnits=m  TranslationThetaOffset=0  TranslationThetaOffsetUnits=deg  RotationMethod=StandardAxis  RotationAngleUnits=deg  RotationStandardAxis=+X  RotationAngle=90  RotationArbitraryAxis=[0 0 1]  FollAlignAxisA=+X  BaseAlignAxisA=+Y  FollAlignAxisB=+Y  BaseAlignAxisB=+Z  RotationSequenceAxes=FollowerAxes  RotationSequence=XYX  RotationSequenceAngles=[0 0 0]  RotationSequenceAnglesUnits=deg  RotationMatrix=[1 0 0; 0 1 0; 0 0 1]  Quaternion=[1 0 0 0]
  W : PMIOPort  Side=Right
  connections:
  Profile Left/RConn1 -- Transform Z to Y Left/RConn1
  Transform Road/LConn1 -- W/RConn1
  Transform Left Profile/LConn1 -- Transform Right Profile/LConn1 -- Transform Road/RConn1
  Transform Z to Y Left/LConn1 -- Transform Left Profile/RConn1
  Profile Right/RConn1 -- Transform Z to Y Right/RConn1
  Transform Right Profile/RConn1 -- Transform Z to Y Right/LConn1
